simulink model "PV_MPPT_DesktopSim"  (R2023b)
settings: Solver=ode23tb  StartTime=0.0  StopTime=inf  MaxStep=1e-4  RelTol=1e-3
PreLoadFcn:
  | load('EmulatedPV_LowPowerData.mat');
  | 
  | numIrr = 10;
  | ArrayPower = ArrayCurrent.*ArrayVoltage;
InitFcn:
  | Ts = 1e-4;
  | Tc = Ts;
undefined symbols (not defined in the file): ArrayCurrent, ArrayVoltage, DiscIntNeverNeededParam, Irradiance, Tdata
libraries: spsSeriesRLCBranchLib x27, fl_lib x15, spsMosfetLib x11, ee_lib x11, spsVoltageMeasurementLib x7, spsCurrentMeasurementLib x6, nesl_utility x5, spsDiodeLib x5, spspowerguiLib x4, spsTriangleGeneratorLib x3, spsParallelRLCBranchLib x3, spsGroundLib x2
(part 3 of 3)

== system PV_MPPT_DesktopSim/Subsystem2/Simple Time Delay Sensor  ==
  u : Inport
  1/Tau : Gain  Gain=1/Tau
  Discrete-Time Integrator : DiscreteIntegrator  SampleTime=Ts  ICPrevOutput=DiscIntNeverNeededParam  ICPrevScaledInput=DiscIntNeverNeededParam
  Sum : Sum  Inputs=|+-
  y : Outport  VectorParamsAs1DForOutWhenUnconnected=off
  wires:
  Discrete-Time Integrator/1 -> Sum/2, y/1
  u/1 -> Sum/1
  Sum/1 -> 1/Tau/1
  1/Tau/1 -> Discrete-Time Integrator/1

== system PV_MPPT_DesktopSim/Subsystem2/Simple Time Delay Sensor 1 ==
  u : Inport
  1/Tau : Gain  Gain=1/Tau
  Discrete-Time Integrator : DiscreteIntegrator  SampleTime=Ts  ICPrevOutput=DiscIntNeverNeededParam  ICPrevScaledInput=DiscIntNeverNeededParam
  Sum : Sum  Inputs=|+-
  y : Outport  VectorParamsAs1DForOutWhenUnconnected=off
  wires:
  1/Tau/1 -> Discrete-Time Integrator/1
  Sum/1 -> 1/Tau/1
  u/1 -> Sum/1
  Discrete-Time Integrator/1 -> y/1, Sum/2

== system PV_MPPT_DesktopSim/Subsystem2/Simulink Function1 ==
  DutyConv : TriggerPort  TriggerType=function-call  IsSimulinkFunction=on  FunctionName=DutyConv  FunctionVisibility=scoped  VariantControl=(inherit)
  Constant : Constant  Value=0.1
  Sum : Sum  Inputs=|+-
  x : ArgIn  DisableCoverage=on  ArgumentName=x
  y : ArgOut  DisableCoverage=on  ArgumentName=y
  wires:
  Constant/1 -> Sum/2
  x/1 -> Sum/1
  Sum/1 -> y/1

== system PV_MPPT_DesktopSim/Subsystem3/Simple Time Delay Sensor  ==
  u : Inport
  1/Tau : Gain  Gain=1/Tau
  Discrete-Time Integrator : DiscreteIntegrator  SampleTime=Ts  ICPrevOutput=DiscIntNeverNeededParam  ICPrevScaledInput=DiscIntNeverNeededParam
  Sum : Sum  Inputs=|+-
  y : Outport  VectorParamsAs1DForOutWhenUnconnected=off
  wires:
  Discrete-Time Integrator/1 -> Sum/2, y/1
  u/1 -> Sum/1
  Sum/1 -> 1/Tau/1
  1/Tau/1 -> Discrete-Time Integrator/1

== system PV_MPPT_DesktopSim/Subsystem3/Simple Time Delay Sensor 1 ==
  u : Inport
  1/Tau : Gain  Gain=1/Tau
  Discrete-Time Integrator : DiscreteIntegrator  SampleTime=Ts  ICPrevOutput=DiscIntNeverNeededParam  ICPrevScaledInput=DiscIntNeverNeededParam
  Sum : Sum  Inputs=|+-
  y : Outport  VectorParamsAs1DForOutWhenUnconnected=off
  wires:
  1/Tau/1 -> Discrete-Time Integrator/1
  Sum/1 -> 1/Tau/1
  u/1 -> Sum/1
  Discrete-Time Integrator/1 -> y/1, Sum/2

== system PV_MPPT_DesktopSim/Subsystem4/SPWM Generator1 ==
  Constant : Constant  Value=0
  Constant1 : Constant  Value=0
  Relational Operator : RelationalOperator  OutDataTypeStr=boolean  RndMeth=Simplest  InputSameDT=off
  Relational Operator1 : RelationalOperator  Operator=<=  OutDataTypeStr=boolean  RndMeth=Simplest  InputSameDT=off
  Sine Wave : Sin  Frequency=2*pi*50  SampleTime=1e-6
  Square Wave Generator : SignalGenerator  WaveForm=square  Frequency=50
  Square Wave Generator1 : SignalGenerator  WaveForm=square  Frequency=50
  Switch : Switch  Criteria=u2 > Threshold  SaturateOnIntegerOverflow=off  InputSameDT=off
  Switch1 : Switch  Criteria=u2 > Threshold  SaturateOnIntegerOverflow=off  InputSameDT=off
  Triangle Generator : spsTriangleGeneratorLib/Triangle Generator  Freq=5000  Phase=90  Ts=0
  Out1 : Outport
  Out2 : Outport  Port=2
  wires:
  Constant/1 -> Switch/3
  Triangle Generator/1 -> Relational Operator/2, Relational Operator1/2
  Relational Operator/1 -> Switch1/3
  Sine Wave/1 -> Relational Operator/1, Relational Operator1/1
  Switch/1 -> Out2/1
  Square Wave Generator/1 -> Switch/2
  Square Wave Generator1/1 -> Switch1/2
  Constant1/1 -> Switch1/1
  Relational Operator1/1 -> Switch/1
  Switch1/1 -> Out1/1

== system PV_MPPT_DesktopSim/Subsystem4/SPWM Generator2 ==
  Constant : Constant  Value=0
  Constant1 : Constant  Value=0
  Relational Operator : RelationalOperator  OutDataTypeStr=boolean  RndMeth=Simplest  InputSameDT=off
  Relational Operator1 : RelationalOperator  Operator=<=  OutDataTypeStr=boolean  RndMeth=Simplest  InputSameDT=off
  Sine Wave : Sin  Frequency=2*pi*50  SampleTime=1e-6
  Square Wave Generator : SignalGenerator  WaveForm=square  Frequency=50
  Square Wave Generator1 : SignalGenerator  WaveForm=square  Frequency=50
  Switch : Switch  Criteria=u2 > Threshold  SaturateOnIntegerOverflow=off  InputSameDT=off
  Switch1 : Switch  Criteria=u2 > Threshold  SaturateOnIntegerOverflow=off  InputSameDT=off
  Triangle Generator : spsTriangleGeneratorLib/Triangle Generator  Freq=5000  Phase=90  Ts=0
  Out1 : Outport
  Out2 : Outport  Port=2
  wires:
  Constant/1 -> Switch/3
  Triangle Generator/1 -> Relational Operator/2, Relational Operator1/2
  Relational Operator/1 -> Switch1/3
  Sine Wave/1 -> Relational Operator/1, Relational Operator1/1
  Switch/1 -> Out2/1
  Square Wave Generator/1 -> Switch/2
  Square Wave Generator1/1 -> Switch1/2
  Constant1/1 -> Switch1/1
  Relational Operator1/1 -> Switch/1
  Switch1/1 -> Out1/1

== matlab function PV_MPPT_DesktopSim/MATLAB Function ==
  settings: updateMethod=DISCRETE
  data: Vpv input; Ipv input; ArrayPower parameter; ArrayVoltage parameter; numIrr parameter
function plotPower(Vpv,Ipv, ArrayPower,ArrayVoltage, numIrr)

    persistent irrPlot powerPlot
%     coder.extrinsic('legend');    
    
    if isempty(irrPlot)
        
        idx = 1:find(ArrayPower(:,numIrr) > 0,1,'last')+2;
                        
        figure(1);
        irrPlot = plot(ArrayVoltage(idx),ArrayPower(idx,1:numIrr)); hold on;
        grid on;
        
        xlabel('PV Voltage [V]');
        ylabel('PV Power [W]');
        title('PV Power Output');
        
        powerPlot = plot(Vpv,Vpv*Ipv,'ro'); 
%         legend('50 W/m^2','100 W/m^2','150 W/m^2','200 W/m^2','250 W/m^2','300 W/m^2',...
%             '350 W/m^2','400 W/m^2','450 W/m^2','500 W/m^2','PV Power');
        hold off;
        
    else 
        set(powerPlot,'XData',Vpv,'YData',Vpv*Ipv);
    end
    
end

== stateflow chart PV_MPPT_DesktopSim/MPPT and Boost Controllers/Perturb and Observe MPPT ==
  state DisableMPPT
    during:
    Vref = VrefCmd;
    Vref_prev = VrefCmd;
  state EnableMPPT
    state Compute_Power
      entry:
      P = V*I;
    state Calculate_Difference
      entry:
      deltaP = P - Pprev;
      deltaV = V - Vprev;
    state Decrement_Vref
      entry:
      Vref = Vref_prev - delV;
    state Increment_Vref
      entry:
      Vref = Vref_prev + delV;
    state Save_PreviousValues
      entry:
      Pprev = P; Vprev = V;
    state Clamp_VrefMax
      entry:
      Vref = VrefMax;
    state Clamp_VrefMin
      entry:
      Vref = VrefMin;
    (default) -> Compute_Power
    (junction 76) -> Compute_Power
    (junction 53) -> (junction 76) : {Vref_prev = Vref;}
    Compute_Power -> Calculate_Difference
    Calculate_Difference -> (junction 13) [order 1] : [deltaP < 0]
    Calculate_Difference -> (junction 14) [order 2] : [deltaP >= 0]
    (junction 13) -> Increment_Vref [order 2] : [deltaV < 0]
    (junction 14) -> Decrement_Vref [order 1] : [deltaV <= 0]
    (junction 13) -> Decrement_Vref [order 1] : [deltaV >= 0]
    (junction 14) -> Increment_Vref [order 2] : [deltaV > 0]
    Decrement_Vref -> Save_PreviousValues
    Increment_Vref -> Save_PreviousValues
    Save_PreviousValues -> (junction 53) [order 3]
    (junction 73) -> (junction 53)
    Save_PreviousValues -> Clamp_VrefMax [order 1] : [Vref >= VrefMax]
    Save_PreviousValues -> Clamp_VrefMin [order 2] : [Vref <= VrefMin]
    Clamp_VrefMax -> (junction 70)
    Clamp_VrefMin -> (junction 50)
    (junction 70) -> (junction 50)
    (junction 50) -> (junction 73)
  (default) -> DisableMPPT
  (junction 91) -> DisableMPPT
  EnableMPPT -> (junction 91) : [MPPT ~= 1]
  DisableMPPT -> EnableMPPT : [MPPT == 1]
  data: P local double =0; k local double =0; Psum local double =0; Vsum local double =0; Vavg local double =0; Pavg local double =0; deltaP local double =0; Pprev local double =0; Vprev local double =0; deltaV local double =0; Vref output double =5; Vref_prev local double =5; VrefMax constant double =28; VrefMin constant double =1; V input double; I input double; VrefCmd input double; MPPT input double; delV input double
  events: event input RISING_EDGE_EVENT
